simulink model "twj_test"  (R2024a)
settings: Solver=FixedStepDiscrete  StartTime=0.0  StopTime=10.0  FixedStep=TsBSP  RelTol=1e-3
libraries: simulink x1
settings Model: DataDictionary=twj.sldd  Creator=chaoli_wanjietian  LastModifiedBy=chaoli_wanjietian

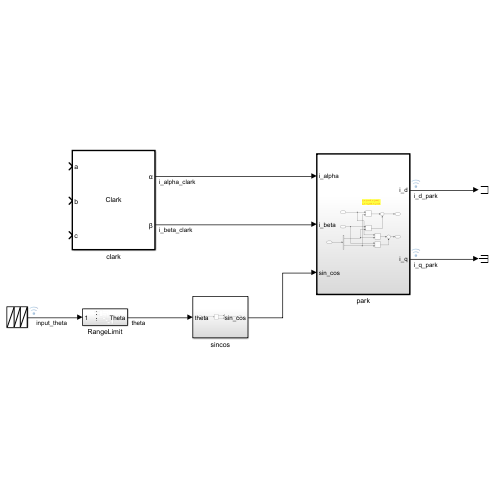
[thumbnail: Simulink's stored preview of the top-level diagram]
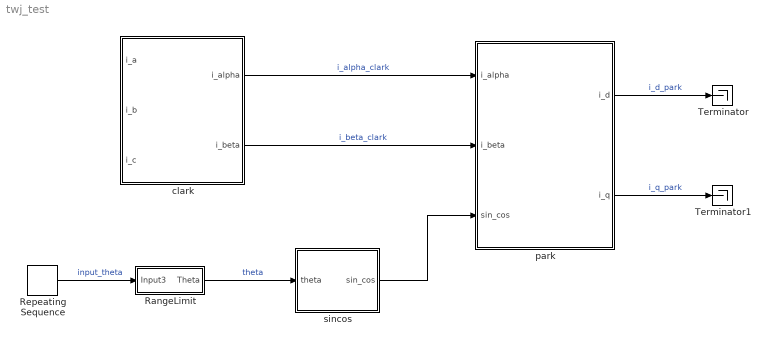
== system twj_test ==
  RangeLimit : Subsystem
  Repeating Sequence : simulink/Sources/Repeating Sequence  rep_seq_t=[0 10]  rep_seq_y=[0 2*pi]
  Terminator : Terminator
  Terminator1 : Terminator
  clark : Subsystem  TreatAsAtomicUnit=on
      mask Display:
      | port_label('input',1,'a','texmode','on');
      | port_label('input',2,'b','texmode','on');
      | port_label('input',3,'c','texmode','on');
      | 
      | port_label('output',1,'\alpha','texmode','on');
      | port_label('output',2,'\beta','texmode','on');
      | 
      | fprintf('Clark');
  park : Subsystem  TreatAsAtomicUnit=on
  sincos : Subsystem
  wires:
  clark/2(i_beta) -> park/2(i_beta)  "i_beta_clark"
  clark/1(i_alpha) -> park/1(i_alpha)  "i_alpha_clark"
  RangeLimit/1(Theta) -> sincos/1(theta)  "theta"
  sincos/1(sin_cos) -> park/3(sin_cos)
  Repeating Sequence/1 -> RangeLimit/1(Input3)  "input_theta"
  park/1(i_d) -> Terminator/1  "i_d_park"
  park/2(i_q) -> Terminator1/1  "i_q_park"

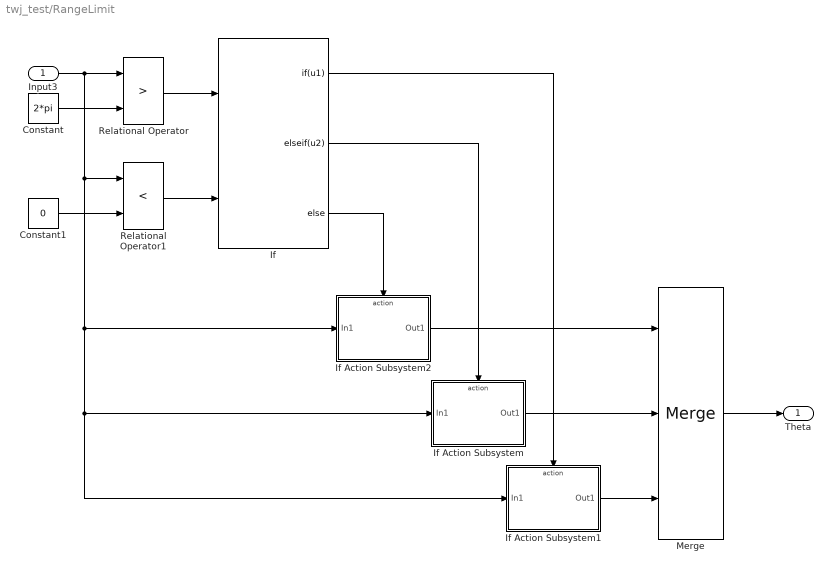
== system twj_test/RangeLimit ==
  Input3 : Inport
  Constant : Constant  Value=2*pi  OutDataTypeStr=double  SampleTime=-1
  Constant1 : Constant  Value=0  OutDataTypeStr=double  SampleTime=-1
  If : If  NumInputs=2  IfExpression=u1  ElseIfExpressions=u2
  If Action Subsystem : Subsystem  TreatAsAtomicUnit=on
  If Action Subsystem1 : Subsystem  TreatAsAtomicUnit=on
  If Action Subsystem2 : Subsystem  TreatAsAtomicUnit=on
  Merge : Merge  Inputs=3
  Relational Operator : RelationalOperator  Operator=>  OutDataTypeStr=boolean  RndMeth=Simplest  InputSameDT=off
  Relational Operator1 : RelationalOperator  Operator=<  OutDataTypeStr=boolean  RndMeth=Simplest  InputSameDT=off
  Theta : Outport
  wires:
  Relational Operator/1 -> If/1
  Constant/1 -> Relational Operator/2
  Constant1/1 -> Relational Operator1/2
  Input3/1 -> Relational Operator1/1, If Action Subsystem2/1(In1), If Action Subsystem1/1(In1), If Action Subsystem/1(In1), Relational Operator/1
  Relational Operator1/1 -> If/2
  Merge/1 -> Theta/1
  If/3 -> If Action Subsystem2/Action
  If/2 -> If Action Subsystem/Action
  If/1 -> If Action Subsystem1/Action
  If Action Subsystem2/1(Out1) -> Merge/1
  If Action Subsystem/1(Out1) -> Merge/2
  If Action Subsystem1/1(Out1) -> Merge/3

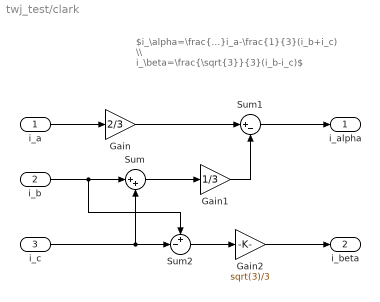
== system twj_test/clark ==
  note: $i_\alpha=\frac{2}{3}i_a-\frac{1}{3}(i_b+i_c) \\ i_\beta=\frac{\sqrt{3}}{3}(i_b-i_c)$
  i_a : Inport
  i_b : Inport  Port=2
  i_c : Inport  Port=3
  Gain : Gain  Gain=2/3
  Gain1 : Gain  Gain=1/3
  Gain2 : Gain  Gain=sqrt(3)/3
  Sum : Sum  Inputs=|++
  Sum1 : Sum  Inputs=|+-
  Sum2 : Sum  Inputs=+-|
  i_alpha : Outport
  i_beta : Outport  Port=2
  wires:
  i_b/1 -> Sum2/1, Sum/1
  Sum/1 -> Gain1/1
  i_c/1 -> Sum2/2, Sum/2
  i_a/1 -> Gain/1
  Gain/1 -> Sum1/1
  Gain1/1 -> Sum1/2
  Sum1/1 -> i_alpha/1
  Sum2/1 -> Gain2/1
  Gain2/1 -> i_beta/1

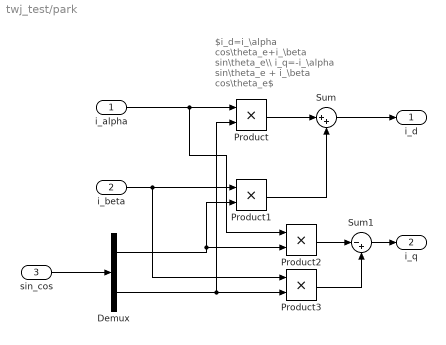
== system twj_test/park ==
  note: $i_d=i_\alpha cos\theta_e+i_\beta sin\theta_e\\ i_q=-i_\alpha sin\theta_e + i_\beta cos\theta_e$
  i_alpha : Inport
  i_beta : Inport  Port=2
  sin_cos : Inport  Port=3
  Demux : Demux  Outputs=2
  Product{,1..3} (4 alike) : Product
  Sum : Sum  Inputs=|++
  Sum1 : Sum  Inputs=|-+
  i_d : Outport
  i_q : Outport  Port=2
  wires:
  sin_cos/1 -> Demux/1
  i_alpha/1 -> Product2/1, Product/1
  Demux/2 -> Product/2, Product3/2
  Demux/1 -> Product1/2, Product2/2
  Product/1 -> Sum/1
  Product1/1 -> Sum/2
  Sum/1 -> i_d/1
  i_beta/1 -> Product3/1, Product1/1
  Product2/1 -> Sum1/1
  Product3/1 -> Sum1/2
  Sum1/1 -> i_q/1

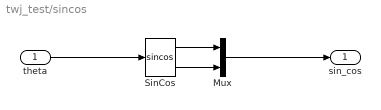
== system twj_test/sincos ==
  theta : Inport
  Mux : Mux  Inputs=2
  SinCos : Trigonometry  Operator=sincos
  sin_cos : Outport
  wires:
  theta/1 -> SinCos/1
  SinCos/2 -> Mux/2
  SinCos/1 -> Mux/1
  Mux/1 -> sin_cos/1

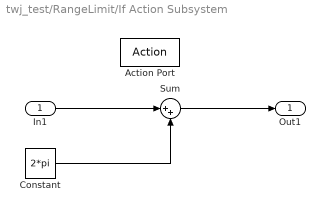
== system twj_test/RangeLimit/If Action Subsystem ==
  In1 : Inport
  Action Port : ActionPort
  Constant : Constant  Value=2*pi  OutDataTypeStr=double  SampleTime=-1
  Sum : Sum  Inputs=|++
  Out1 : Outport
  wires:
  In1/1 -> Sum/1
  Constant/1 -> Sum/2
  Sum/1 -> Out1/1

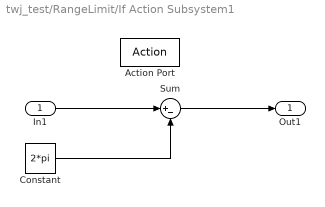
== system twj_test/RangeLimit/If Action Subsystem1 ==
  In1 : Inport
  Action Port : ActionPort
  Constant : Constant  Value=2*pi  OutDataTypeStr=double  SampleTime=-1
  Sum : Sum  Inputs=|+-
  Out1 : Outport
  wires:
  In1/1 -> Sum/1
  Constant/1 -> Sum/2
  Sum/1 -> Out1/1

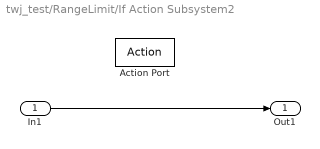
== system twj_test/RangeLimit/If Action Subsystem2 ==
  In1 : Inport
  Action Port : ActionPort
  Out1 : Outport
  wires:
  In1/1 -> Out1/1
